simulink model "one_area_model"  (R2016b)
settings: Solver=VariableStepAuto  StartTime=0.0  StopTime=3000  RelTol=1e-3
values from neighbouring files (symbols this model uses):
  B_freq = 1/S    (= 25)    [run_simulation.m]
  C_p = 0.17    [run_simulation.m]
  D_L = 1/200    (= 0.005)    [run_simulation.m]
  J = [J11 J12(:,idx_pq) J13; J21(idx_pq,:) J22(idx_pq,idx_pq) J23(idx_pq)]    [pf_with_AGC.m]    (also in run_simulation.m = 40)
  S = 0.04    [run_simulation.m]
  T_N = 120    [run_simulation.m]
  T_t = 0    [run_simulation.m]
  w0 = 50    [run_simulation.m]
  W_0 = 0    [run_simulation.m]
settings Model: Creator=dc  LastModifiedBy=dc

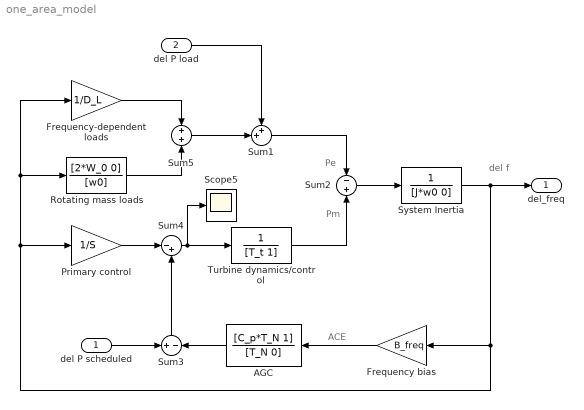
== system one_area_model ==
  note: Pm
  note: Pe
  note: ACE
  note: del f
  del P scheduled : Inport
  del P load : Inport  Port=2
  AGC : TransferFcn  Numerator=[C_p*T_N 1]  Denominator=[T_N 0]
  Frequency bias : Gain  Gain=B_freq
  Frequency-dependent loads : Gain  Gain=1/D_L
  Primary control : Gain  Gain=1/S
  Rotating mass loads : TransferFcn  Numerator=[2*W_0 0]  Denominator=[w0]
  Scope5 : Scope
  Sum1 : Sum  Inputs=++|
  Sum2 : Sum  Inputs=-|+
  Sum3 : Sum  Inputs=+|-
  Sum4 : Sum  Inputs=|-+
  Sum5 : Sum  Inputs=+|+
  System Inertia : TransferFcn  Denominator=[J*w0 0]
  Turbine dynamics/control : TransferFcn  Denominator=[T_t 1]
  del_freq : Outport
  wires:
  Frequency-dependent loads/1 -> Sum5/1
  Rotating mass loads/1 -> Sum5/2
  Sum2/1 -> System Inertia/1
  Turbine dynamics/control/1 -> Sum2/2
  Sum1/1 -> Sum2/1
  System Inertia/1 -> del_freq/1, Rotating mass loads/1, Frequency-dependent loads/1, Primary control/1, Frequency bias/1
  Frequency bias/1 -> AGC/1
  Sum4/1 -> Scope5/1, Turbine dynamics/control/1
  Primary control/1 -> Sum4/1
  Sum3/1 -> Sum4/2
  AGC/1 -> Sum3/2
  Sum5/1 -> Sum1/2
  del P scheduled/1 -> Sum3/1
  del P load/1 -> Sum1/1
